simulink model "ADC_model"  (R2018b)
settings: Solver=VariableStepAuto  StartTime=0.0  StopTime=Endtime  RelTol=1e-3
values from neighbouring files (symbols this model uses):
  alpha_A = (2^n - 1)/(V_A_max - V_A_min)    (= 204.6)    [ADC_sim.m]    (also in controller_sim.m)
  smp = 0.001    [ADC_sim.m]    (also in controller_sim.m; pulse_gen_sim.m = 0.01)
  v_A_d = 1    [ADC_sim.m]    (also in controller_sim.m)
  V_A_max = 5    [ADC_sim.m]    (also in controller_sim.m)
  V_A_min = 0    [ADC_sim.m]    (also in controller_sim.m)
libraries: simulink x1
settings Model: Creator=nharada  LastModifiedBy=nharada

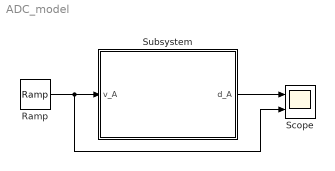
== system ADC_model ==
  Ramp : simulink/Sources/Ramp  slope=v_A_d  start=0  InitialOutput=-5
  Scope : Scope  NumInputPorts=2
  Subsystem : Subsystem
  wires:
  Ramp/1 -> Scope/2, Subsystem/1(v_A)
  Subsystem/1(d_A) -> Scope/1

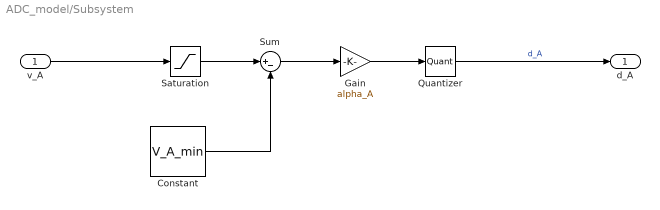
== system ADC_model/Subsystem ==
  v_A : Inport
  Constant : Constant  Value=V_A_min  SampleTime=smp
  Gain : Gain  Gain=alpha_A
  Quantizer : Quantizer  QuantizationInterval=1
  Saturation : Saturate  UpperLimit=V_A_max  LowerLimit=V_A_min
  Sum : Sum  Inputs=|+-
  d_A : Outport
  wires:
  Saturation/1 -> Sum/1
  Constant/1 -> Sum/2
  Sum/1 -> Gain/1
  Gain/1 -> Quantizer/1
  v_A/1 -> Saturation/1
  Quantizer/1 -> d_A/1  "d_A"
